simulink model "Drv001"  (Simulink 8.3)
settings: Solver=ode45  StartTime=0.0  StopTime=10.0  RelTol=1e-3
model workspace (MAT data in the model file):
  pDrv : struct (value not decoded)
settings Model: Creator=swami  LastModifiedBy=swami
settings DataIOCC: SignalLoggingSaveFormat=Dataset
settings DebuggingCC: UnderspecifiedInitializationDetection=Simplified  StateNameClashWarn=none
settings GRTTargetCC: CombineOutputUpdateFcns=on  GRTInterface=off

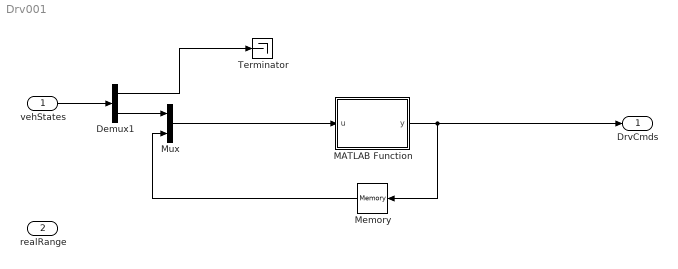
== system Drv001 ==
  vehStates : Inport
  realRange : Inport  Port=2
  Demux1 : Demux  Outputs=2
  MATLAB Function : MATLAB Function  TreatAsAtomicUnit=on
  Memory : Memory
  Mux : Mux  Inputs=2
  Terminator : Terminator
  DrvCmds : Outport
  wires:
  MATLAB Function/1(y) -> Memory/1, DrvCmds/1
  vehStates/1 -> Demux1/1
  Demux1/1 -> Terminator/1
  Demux1/2 -> Mux/1
  Mux/1 -> MATLAB Function/1(u)
  Memory/1 -> Mux/2

== matlab function MATLAB Function ==
  data: u input double; y output double; pDrv parameter double
function y = fcn(u,pDrv)
y = [0,0,0,0];
spd = u(1);
CCSw = u(4);
CCSetPt = pDrv.CCSetPt;
%#codegen
if (spd< CCSetPt && CCSw<0.5)
    y(1) = 0.0; %brake
    y(2) = 1.0; %throttle
    y(3) = 0.0; %Cruise Control Switch
    y(4) = 0.0;
else
    y(1) = 0.0;
    y(2) = 0.0;
    y(3) = 1.0;
    y(4) = CCSetPt;
end
